simulink model "iir_example_sim"  (R2014a)
settings: Solver=VariableStepDiscrete  StartTime=0.0  StopTime=1  RelTol=1e-3
values from neighbouring files (symbols this model uses):
  dt = 1/Fs    (= 2.26757369615e-05)    [iir_matlab_to_C.m]    (also in iir_simulink_example.m = 0.0002)
  Fn1 = 1000    [iir_matlab_to_C.m]    (also in iir_simulink_example.m = 100)
  Fn2 = 10000    [iir_matlab_to_C.m]    (also in iir_simulink_example.m = 500)
undefined symbols (not defined in the file or in its folder): dfilt
libraries: dspsrcs4 x2, dsparch4 x1
settings Model: Creator=rodralez  LastModifiedBy=rodralez

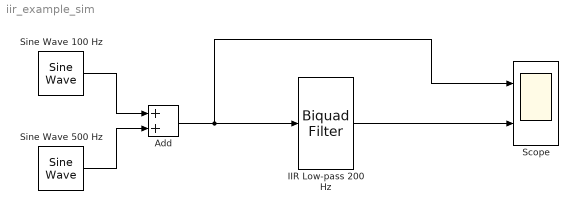
== system iir_example_sim ==
  Add : Sum
  IIR Low-pass 200 Hz : dsparch4/Biquad Filter  IIRFiltStruct=Direct form II transposed  CoeffSource=Specify via dialog  BiQuadCoeffs=Hd.sosMatrix  a0Flag=Warning  IC=0  ICnum=0  ICden=0  InputProcessing=Inherited (this choice will be removed - see release notes)  denAccumFracLength=30  denProdOutputFracLength=30  secondMemoryFracLength=15  roundingMode=Nearest  overflowMode=on  ScaleValues=Hd.ScaleValues  optimizeScaleValues=on  ScaleValueMode=Specify via input port (g)  scaleValueFracLength=14  FilterSource=Specify via dialog  dfiltObjectName=dfilt.df2tsos([1 0.3 0.4],[1 0.1 0.2])
  Scope : Scope  NumInputPorts=2
      settings: TimeRange=1  YMin=-5~-5  YMax=5~5
  Sine Wave 100 Hz : dspsrcs4/Sine Wave  Amplitude=1  Frequency=Fn1  Phase=0  SampleMode=Discrete  OutComplex=Real  CompMethod=Trigonometric fcn  TableSize=Speed  SampleTime=dt  SamplesPerFrame=1  ResetState=Restart at time zero  dataType=single  wordLen=16  udDataType=sfix(16)  fracBitsMode=Best precision  numFracBits=15  OutDataTypeStr=single  LastOutDataTypeStr=single
  Sine Wave 500 Hz : dspsrcs4/Sine Wave  Amplitude=1  Frequency=Fn2  Phase=0  SampleMode=Discrete  OutComplex=Real  CompMethod=Trigonometric fcn  TableSize=Speed  SampleTime=dt  SamplesPerFrame=1  ResetState=Restart at time zero  dataType=single  wordLen=16  udDataType=sfix(16)  fracBitsMode=Best precision  numFracBits=15  OutDataTypeStr=single  LastOutDataTypeStr=single
  wires:
  Sine Wave 100 Hz/1 -> Add/1
  Sine Wave 500 Hz/1 -> Add/2
  IIR Low-pass 200 Hz/1 -> Scope/2
  Add/1 -> IIR Low-pass 200 Hz/1, Scope/1
